simulink model "flamingo_link"  (R2019a)
settings: Solver=FixedStepDiscrete  StartTime=0.0  StopTime=inf  FixedStep=1/500  RelTol=1e-3
PreLoadFcn:
  | x_setpoint_NED = 0;
  | y_setpoint_NED = 0;
  | z_setpoint_NED = 0;
  | vx_setpoint_NED = 0;
  | vy_setpoint_NED = 0;
  | vz_setpoint_NED = 0;
  | afx_setpoint_NED = 0;
  | afy_setpoint_NED = 0;
  | afz_setpoint_NED = 0;
  | yaw_setpoint_NED = 0;
  | yawrate_setpoint_NED = 0;
  | selected_mission = 0;
  | reboot_cmd = 0;
  | return_com = 0;
  | takeoff_com = 0;
  | mission_com = 0;
  | hold_com = 0;
  | land_com = 0;
  | direct_com = 0;
  | origin_com = 0;
InitFcn:
  | x_setpoint_NED = 0;
  | y_setpoint_NED = 0;
  | z_setpoint_NED = 0;
  | vx_setpoint_NED = 0;
  | vy_setpoint_NED = 0;
  | vz_setpoint_NED = 0;
  | afx_setpoint_NED = 0;
  | afy_setpoint_NED = 0;
  | afz_setpoint_NED = 0;
  | yaw_setpoint_NED = 0;
  | yawrate_setpoint_NED = 0;
  | selected_mission = 0;
  | reboot_cmd = 0;
  | return_com = 0;
  | takeoff_com = 0;
  | mission_com = 0;
  | hold_com = 0;
  | land_com = 0;
  | direct_com = 0;
  | origin_com = 0;
undefined symbols (not defined in the file or in its folder): afx, afy, afz, command, confirmation, coordinate_frame, f, Object1, Object2, origin_pos, param1, param2, param3, param4, param5, param6, param7, pitch, roll, Standard_Devices, target_component, target_system, time_boot_ms, time_usec, type_mask, UDP_Protocol, vx, vy, vz, x, y, yaw, yaw_rate, z
libraries: simulink x11, sldrtlib x4, instrumentlib x1
settings Model: Creator=Admin  LastModifiedBy=viconadmin
settings SolverCC: PositivePriorityOrder=on  AutoInsertRateTranBlk=on  InsertRTBMode=Never (minimum delay)
settings DebuggingCC: ReadBeforeWriteMsg=DisableAll  WriteAfterWriteMsg=DisableAll  WriteAfterReadMsg=DisableAll  MultiTaskDSMMsg=none  ArithmeticOperatorsInVariantConditions=warning
settings ModelReferenceCC: UpdateModelReferenceTargets=IfOutOfDate
settings SFSimCC: SFSimEcho=off  SimUseLocalCustomCode=off
settings RTWCC: SystemTargetFile=sldrt.tlc  TemplateMakefile=sldrt.tmf  Description=Simulink Desktop Real-Time  RTWUseLocalCustomCode=off  RTWCompilerOptimization=on
settings CodeAppCC: MaxIdLength=95  StateflowObjectComments=on
settings SimulinkDesktopRealTimeCC: TargetPreCompLibLocation=C:\Program Files\MATLAB\R2019a\toolbox\sldrt\lib\win64  PreserveStateflowLocalDataDimensions=off

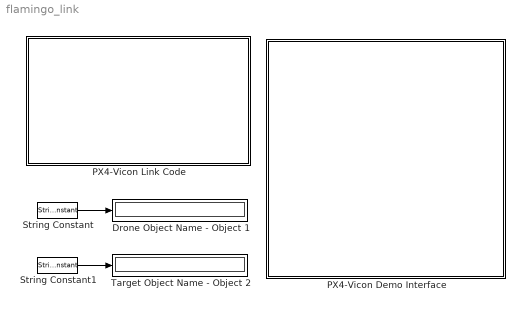
== system flamingo_link ==
  Drone Object Name - Object 1 : Display
  PX4-Vicon Demo Interface : Subsystem
  PX4-Vicon Link Code : Subsystem
  String Constant : StringConstant  String=Object1
  String Constant1 : StringConstant  String=Object2
  Target Object Name - Object 2 : Display
  wires:
  String Constant/1 -> Drone Object Name - Object 1/1
  String Constant1/1 -> Target Object Name - Object 2/1

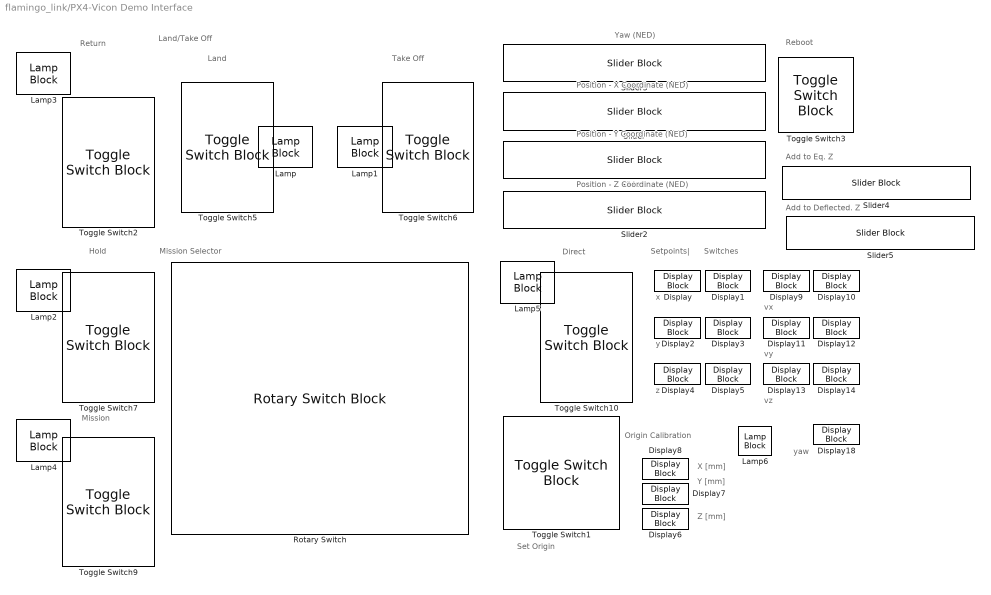
== system flamingo_link/PX4-Vicon Demo Interface ==
  note: Position - X Coordinate (NED)
  note: Position - Y Coordinate (NED)
  note: Position - Z Coordinate (NED)
  note: Yaw (NED)
  note: Mission Selector
  note: Setpoints|
  note: Switches
  note: x
  note: y
  note: z
  note: yaw
  note: Mission
  note: Direct
  note: Hold
  note: Return
  note: Take Off
  note: Land
  note: Land/Take Off
  note: Set Origin
  note: X [mm]
  note: Y [mm]
  note: Z [mm]
  note: Origin Calibration
  note: Reboot
  note: vz
  note: vx
  note: vy
  note: Add to Eq. Z
  note: Add to Deflected. Z
  Display{,1..14,18} (16 alike) : DisplayBlock  LabelPosition=Hide  Format=short
  Lamp{,1..6} (7 alike) : LampBlock  LabelPosition=Hide
  Rotary Switch : RotarySwitchBlock  LabelPosition=Hide
      settings: Values={{'Hold Origin', 'Pulses X', 'Circle'}, [0 1 2]}
  Slider : SliderBlock  LabelPosition=Hide  ScaleMin=-0.5  ScaleMax=0.5  TickInterval=0.10000000000000001
  Slider1 : SliderBlock  LabelPosition=Hide  ScaleMin=-0.5  ScaleMax=0.5  TickInterval=0.10000000000000001
  Slider2 : SliderBlock  LabelPosition=Hide  ScaleMin=-1.5  ScaleMax=0  TickInterval=0.10000000000000001
  Slider3 : SliderBlock  LabelPosition=Hide  ScaleMin=-3  ScaleMax=3
  Slider4 : SliderBlock  LabelPosition=Hide  ScaleMin=-0.14999999999999999  ScaleMax=0.14999999999999999
  Slider5 : SliderBlock  LabelPosition=Hide  ScaleMin=-0.14999999999999999  ScaleMax=0.14999999999999999
  Toggle Switch{1..3,5..7,9..10} (8 alike) : ToggleSwitchBlock  LabelPosition=Hide

== system flamingo_link/PX4-Vicon Link Code ==
  note: MAVLink PX4 Interface Telemetry
  note: MAVLink PX4 Interface Motion Capture
  Data Manipulation : Subsystem
  Decode PX4  Telemetry Data - MAVLink : S-Function  FunctionName=sfun_decode_mavlink  SFunctionDeploymentMode=off  EnableBusSupport=off
  Mavlink Encoded - UDP Packet Output : sldrtlib/Packet Output  SampleTime=1/50  MaxMissedTicks=inf  ShowMissedTicks=off  YieldWhenWaiting=off  DrvName=Standard_Devices/UDP_Protocol  DrvAddress=14551  DrvOptions=[0 14556 48 46 48 46 48 46 48 0 0 0 0 0 0 0 0 0 0 0 0 0 0 0 0 0 0 0 0 0 0 0 0 0 0 0 0 0 0 0 0 0 0 0 0 0 0 0 0 0 0 0 0 0 0 0 0 0 0 0 0 0 0 0 0 0 0 0 0 0 0 0 0 0 0 0 0 0 0 0 0 0 0 0 0 0 0 0 0 0 0 0 0 0 0 0 0 0 0 0 0 0 0 0 0 0 0 0 0 0 0 0 0 0 0 0 0 0 0 0 0 0 0 0 0 0 0 0 0 0 0 0 0 0 0 0 0 0 0 0 0 0 0 0 0 0 0 0 0 0 0 0 0 0 0 0 0 0 0 0 0 0 0 0 0 0 0 0 0 0 0 0 0 0 0 0 0 0 0 0 0 0 0 0 0 0 0 0 0 0 0 0 0 0 0 0 0 0 0 0 0 0 0 0 0 0 0 0 0 0 0 0 0 0 0 0 0 0 0 0 0 0 0 0 0 0 0 0 0 0 0 0 0 0 0 0 0 0 0 0 0 0 0 0 0 0 0 0 0 0 0 0 0 0 0 0]  PacketSize=65  DataTypes='65*uint8'  ShowReady=off  ShowError=off  PacketID=1  ByteOrder=1  InitialValue=[]  FinalValue=[]
      settings: AttributesFormatString=UDP Protocol [14551]  SourceProductName=Simulink Desktop Real-Time
  Mavlink Encoded - UDP Packet Output1 : sldrtlib/Packet Output  Priority=10  SampleTime=1/50  MaxMissedTicks=inf  ShowMissedTicks=off  YieldWhenWaiting=off  DrvName=Standard_Devices/UDP_Protocol  DrvAddress=14551  DrvOptions=[0 14556 48 46 48 46 48 46 48 0 0 0 0 0 0 0 0 0 0 0 0 0 0 0 0 0 0 0 0 0 0 0 0 0 0 0 0 0 0 0 0 0 0 0 0 0 0 0 0 0 0 0 0 0 0 0 0 0 0 0 0 0 0 0 0 0 0 0 0 0 0 0 0 0 0 0 0 0 0 0 0 0 0 0 0 0 0 0 0 0 0 0 0 0 0 0 0 0 0 0 0 0 0 0 0 0 0 0 0 0 0 0 0 0 0 0 0 0 0 0 0 0 0 0 0 0 0 0 0 0 0 0 0 0 0 0 0 0 0 0 0 0 0 0 0 0 0 0 0 0 0 0 0 0 0 0 0 0 0 0 0 0 0 0 0 0 0 0 0 0 0 0 0 0 0 0 0 0 0 0 0 0 0 0 0 0 0 0 0 0 0 0 0 0 0 0 0 0 0 0 0 0 0 0 0 0 0 0 0 0 0 0 0 0 0 0 0 0 0 0 0 0 0 0 0 0 0 0 0 0 0 0 0 0 0 0 0 0 0 0 0 0 0 0 0 0 0 0 0 0 0 0 0 0 0 0]  PacketSize=44  DataTypes='44*uint8'  ShowReady=off  ShowError=off  PacketID=1  ByteOrder=1  InitialValue=[]  FinalValue=[]
      settings: AttributesFormatString=UDP Protocol [14551]  SourceProductName=Simulink Desktop Real-Time
  Mavlink Encoded - UDP Packet Output2 : sldrtlib/Packet Output  SampleTime=1/5  MaxMissedTicks=inf  ShowMissedTicks=off  YieldWhenWaiting=off  DrvName=Standard_Devices/UDP_Protocol  DrvAddress=14551  DrvOptions=[0 14556 48 46 48 46 48 46 48 0 0 0 0 0 0 0 0 0 0 0 0 0 0 0 0 0 0 0 0 0 0 0 0 0 0 0 0 0 0 0 0 0 0 0 0 0 0 0 0 0 0 0 0 0 0 0 0 0 0 0 0 0 0 0 0 0 0 0 0 0 0 0 0 0 0 0 0 0 0 0 0 0 0 0 0 0 0 0 0 0 0 0 0 0 0 0 0 0 0 0 0 0 0 0 0 0 0 0 0 0 0 0 0 0 0 0 0 0 0 0 0 0 0 0 0 0 0 0 0 0 0 0 0 0 0 0 0 0 0 0 0 0 0 0 0 0 0 0 0 0 0 0 0 0 0 0 0 0 0 0 0 0 0 0 0 0 0 0 0 0 0 0 0 0 0 0 0 0 0 0 0 0 0 0 0 0 0 0 0 0 0 0 0 0 0 0 0 0 0 0 0 0 0 0 0 0 0 0 0 0 0 0 0 0 0 0 0 0 0 0 0 0 0 0 0 0 0 0 0 0 0 0 0 0 0 0 0 0 0 0 0 0 0 0 0 0 0 0 0 0 0 0 0 0 0 0]  PacketSize=45  DataTypes='45*uint8'  ShowReady=off  ShowError=off  PacketID=1  ByteOrder=1  InitialValue=[]  FinalValue=[]
      settings: AttributesFormatString=UDP Protocol [14551]  SourceProductName=Simulink Desktop Real-Time
  Packet Input : sldrtlib/Packet Input  SampleTime=1/50  MaxMissedTicks=inf  ShowMissedTicks=off  YieldWhenWaiting=off  DrvName=Standard_Devices/UDP_Protocol  DrvAddress=14551  DrvOptions=[0 14556 48 46 48 46 48 46 48 0 0 0 0 0 0 0 0 0 0 0 0 0 0 0 0 0 0 0 0 0 0 0 0 0 0 0 0 0 0 0 0 0 0 0 0 0 0 0 0 0 0 0 0 0 0 0 0 0 0 0 0 0 0 0 0 0 0 0 0 0 0 0 0 0 0 0 0 0 0 0 0 0 0 0 0 0 0 0 0 0 0 0 0 0 0 0 0 0 0 0 0 0 0 0 0 0 0 0 0 0 0 0 0 0 0 0 0 0 0 0 0 0 0 0 0 0 0 0 0 0 0 0 0 0 0 0 0 0 0 0 0 0 0 0 0 0 0 0 0 0 0 0 0 0 0 0 0 0 0 0 0 0 0 0 0 0 0 0 0 0 0 0 0 0 0 0 0 0 0 0 0 0 0 0 0 0 0 0 0 0 0 0 0 0 0 0 0 0 0 0 0 0 0 0 0 0 0 0 0 0 0 0 0 0 0 0 0 0 0 0 0 0 0 0 0 0 0 0 0 0 0 0 0 0 0 0 0 0 0 0 0 0 0 0 0 0 0 0 0 0 0 0 0 0 0 0]  PacketSize=280  DataTypes='280*uint8'  ShowReady=off  ShowError=off  PacketID=1  ByteOrder=1  ShowTimestamp=off
      settings: AttributesFormatString=UDP Protocol [14551]  SourceProductName=Simulink Desktop Real-Time
  Rate Transition : RateTransition
  Rate Transition1 : RateTransition
  Rate Transition2 : RateTransition
  Vicon Stream - UDP Packet Receive : instrumentlib/UDP Receive  Priority=10  Host=localhost  Port=9090  LocalPort=51001  EnablePortSharing=off  GetLatestData=off  DataSize=256  DataType=uint8  ASCIIFormatting=%f,  Terminator=LF  ByteOrder=BigEndian  EnableBlockingMode=off  Timeout=inf  SampleTime=-1  LocalAddress=0.0.0.0
      settings: SourceProductName=Instrument Control Toolbox
  Visualize Telemetry Data : Subsystem
  wires:
  Rate Transition/1 -> Mavlink Encoded - UDP Packet Output/1
  Packet Input/1 -> Decode PX4  Telemetry Data - MAVLink/1
  Vicon Stream - UDP Packet Receive/1 -> Data Manipulation/1(vicon_data_input)
  Vicon Stream - UDP Packet Receive/2 -> Data Manipulation/2(status)
  Decode PX4  Telemetry Data - MAVLink/2 -> Visualize Telemetry Data/2(telemetry_attitude)
  Data Manipulation/2(Encoded_Mocap_Output) -> Rate Transition1/1
  Decode PX4  Telemetry Data - MAVLink/1 -> Visualize Telemetry Data/1(msg_heartbeat)
  Visualize Telemetry Data/1(FLAG_ARMED) -> Data Manipulation/3(FLAG_ARMED)
  Data Manipulation/1(Encoded_Setpoints_Output) -> Rate Transition/1
  Data Manipulation/3(Encoded_Reboot_Output) -> Rate Transition2/1
  Rate Transition1/1 -> Mavlink Encoded - UDP Packet Output1/1
  Rate Transition2/1 -> Mavlink Encoded - UDP Packet Output2/1

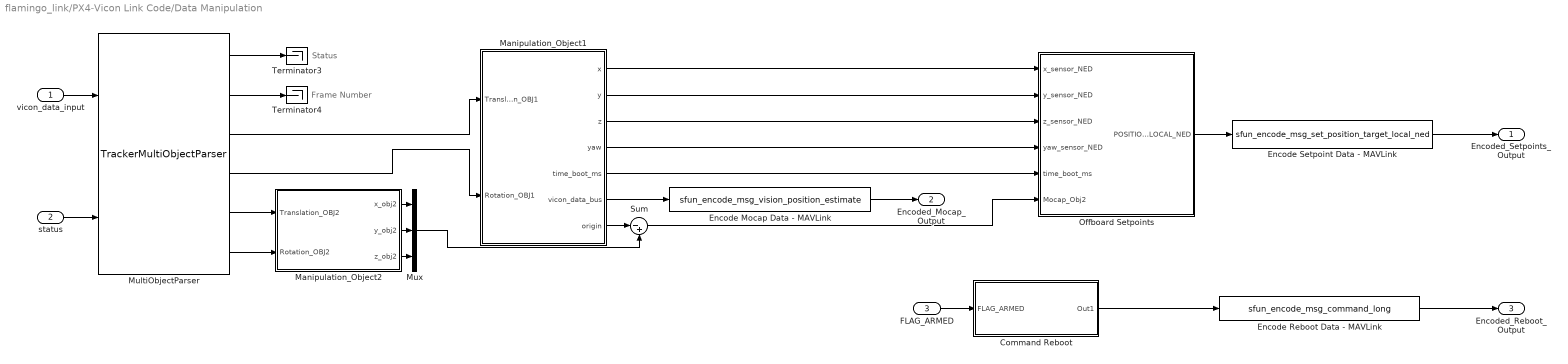
== system flamingo_link/PX4-Vicon Link Code/Data Manipulation ==
  note: Status
  note: Frame Number
  vicon_data_input : Inport
  status : Inport  Port=2
  FLAG_ARMED : Inport  Port=3
  Command Reboot : Subsystem
  "Encode Mocap Data - MAVLink " : S-Function  Priority=10  FunctionName=sfun_encode_msg_vision_position_estimate  SFunctionDeploymentMode=off  EnableBusSupport=off
  Encode Reboot Data - MAVLink : S-Function  FunctionName=sfun_encode_msg_command_long  SFunctionDeploymentMode=off  EnableBusSupport=off
  Encode Setpoint Data - MAVLink : S-Function  FunctionName=sfun_encode_msg_set_position_target_local_ned  SFunctionDeploymentMode=off  EnableBusSupport=off
  Manipulation_Object1 : Subsystem  Priority=10
  Manipulation_Object2 : Subsystem
  MultiObjectParser : S-Function  Tag=Data_Parser_Multi  Priority=10  FunctionName=TrackerMultiObjectParser  Parameters=Object1,Object2  SFunctionModules=TrackerMultiObjectParser  SFunctionDeploymentMode=off  EnableBusSupport=off
      settings: AttributesFormatString=Data_Parser_Multi
  Mux : Mux  Inputs=3
  Offboard Setpoints : Subsystem
  Sum : Sum  Inputs=|-+
  Terminator3 : Terminator
  Terminator4 : Terminator
  Encoded_Setpoints_Output : Outport
  Encoded_Mocap_Output : Outport  Port=2
  Encoded_Reboot_Output : Outport  Port=3
  wires:
  MultiObjectParser/3 -> Manipulation_Object1/1(Translation_OBJ1)
  MultiObjectParser/2 -> Terminator4/1
  Manipulation_Object1/1(x) -> Offboard Setpoints/1(x_sensor_NED)
  MultiObjectParser/1 -> Terminator3/1
  Manipulation_Object1/6(vicon_data_bus) -> "Encode Mocap Data - MAVLink "/1
  MultiObjectParser/5 -> Manipulation_Object2/1(Translation_OBJ2)
  MultiObjectParser/6 -> Manipulation_Object2/2(Rotation_OBJ2)
  MultiObjectParser/4 -> Manipulation_Object1/2(Rotation_OBJ1)
  Manipulation_Object1/4(yaw) -> Offboard Setpoints/4(yaw_sensor_NED)
  status/1 -> MultiObjectParser/2
  Manipulation_Object1/3(z) -> Offboard Setpoints/3(z_sensor_NED)
  Manipulation_Object1/2(y) -> Offboard Setpoints/2(y_sensor_NED)
  "Encode Mocap Data - MAVLink "/1 -> Encoded_Mocap_Output/1
  vicon_data_input/1 -> MultiObjectParser/1
  Manipulation_Object1/5(time_boot_ms) -> Offboard Setpoints/5(time_boot_ms)
  Offboard Setpoints/1(POSITION_TARGET_LOCAL_NED) -> Encode Setpoint Data - MAVLink/1
  Encode Setpoint Data - MAVLink/1 -> Encoded_Setpoints_Output/1
  Mux/1 -> Sum/2
  Command Reboot/1(Out1) -> Encode Reboot Data - MAVLink/1
  FLAG_ARMED/1 -> Command Reboot/1(FLAG_ARMED)
  Encode Reboot Data - MAVLink/1 -> Encoded_Reboot_Output/1
  Manipulation_Object2/3(z_obj2) -> Mux/3
  Manipulation_Object2/2(y_obj2) -> Mux/2
  Manipulation_Object2/1(x_obj2) -> Mux/1
  Manipulation_Object1/7(origin) -> Sum/1
  Sum/1 -> Offboard Setpoints/6(Mocap_Obj2)

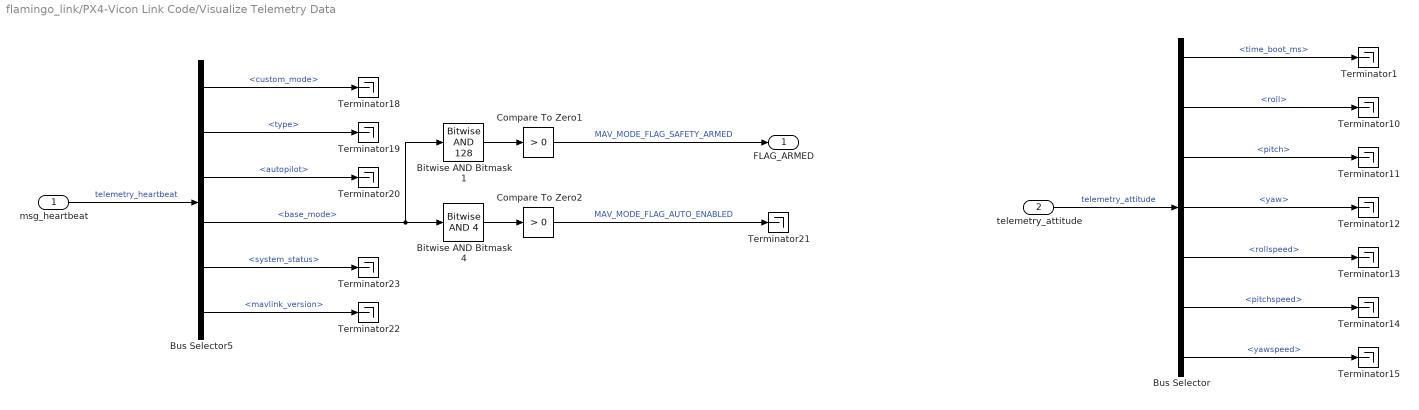
== system flamingo_link/PX4-Vicon Link Code/Visualize Telemetry Data ==
  msg_heartbeat : Inport
  telemetry_attitude : Inport  Port=2
  Bitwise AND Bitmask 1 : simulink/Logic and Bit Operations/Bitwise Operator  logicop=AND  UseBitMask=on  BitMask=128  BitMaskRealWorld=Stored Integer
  Bitwise AND Bitmask 4 : simulink/Logic and Bit Operations/Bitwise Operator  logicop=AND  UseBitMask=on  BitMask=4  BitMaskRealWorld=Stored Integer
  Bus Selector : BusSelector  OutputSignals=time_boot_ms,roll,pitch,yaw,rollspeed,pitchspeed,yawspeed
  Bus Selector5 : BusSelector  OutputSignals=custom_mode,type,autopilot,base_mode,system_status,mavlink_version
  Compare To Zero1 : simulink/Logic and Bit Operations/Compare To Zero  relop=>  OutDataTypeStr=boolean
  Compare To Zero2 : simulink/Logic and Bit Operations/Compare To Zero  relop=>  OutDataTypeStr=boolean
  Terminator{1,10..15,18..23} (13 alike) : Terminator
  FLAG_ARMED : Outport
  wires:
  Bus Selector/7 -> Terminator15/1  "<yawspeed>"
  Bus Selector/5 -> Terminator13/1  "<rollspeed>"
  Bus Selector/2 -> Terminator10/1  "<roll>"
  Bus Selector/1 -> Terminator1/1  "<time_boot_ms>"
  Bus Selector/4 -> Terminator12/1  "<yaw>"
  Bus Selector/3 -> Terminator11/1  "<pitch>"
  Bus Selector/6 -> Terminator14/1  "<pitchspeed>"
  telemetry_attitude/1 -> Bus Selector/1  "telemetry_attitude"
  Bus Selector5/4 -> Bitwise AND Bitmask 1/1, Bitwise AND Bitmask 4/1  "<base_mode>"
  Bitwise AND Bitmask 4/1 -> Compare To Zero2/1
  Bitwise AND Bitmask 1/1 -> Compare To Zero1/1
  Bus Selector5/3 -> Terminator20/1  "<autopilot>"
  Compare To Zero1/1 -> FLAG_ARMED/1  "MAV_MODE_FLAG_SAFETY_ARMED"
  Bus Selector5/6 -> Terminator22/1  "<mavlink_version>"
  Bus Selector5/5 -> Terminator23/1  "<system_status>"
  Bus Selector5/2 -> Terminator19/1  "<type>"
  Bus Selector5/1 -> Terminator18/1  "<custom_mode>"
  msg_heartbeat/1 -> Bus Selector5/1  "telemetry_heartbeat"
  Compare To Zero2/1 -> Terminator21/1  "MAV_MODE_FLAG_AUTO_ENABLED"

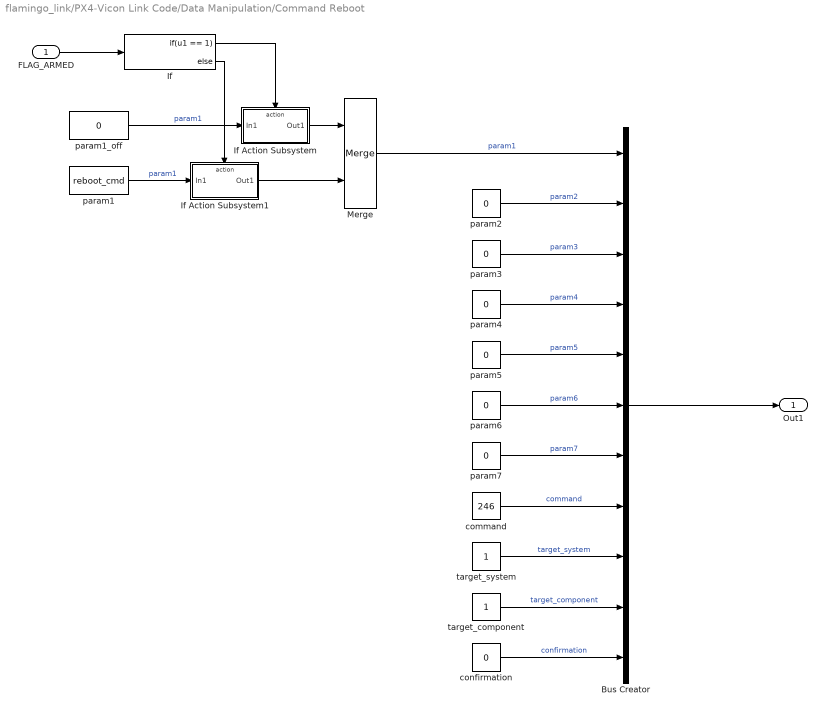
== system flamingo_link/PX4-Vicon Link Code/Data Manipulation/Command Reboot ==
  FLAG_ARMED : Inport
  Bus Creator : BusCreator  Inputs=param1,param2,param3,param4,param5,param6,param7,command,target_system,target_component,confirmation  OutDataTypeStr=Bus: mavlink_command_long_t
  If : If  IfExpression=u1 == 1
  If Action Subsystem : Subsystem  TreatAsAtomicUnit=on
  If Action Subsystem1 : Subsystem  TreatAsAtomicUnit=on
  Merge : Merge
  command : Constant  Value=246  OutDataTypeStr=uint16
  confirmation : Constant  Value=0  OutDataTypeStr=uint8
  param1 : Constant  Value=reboot_cmd  OutDataTypeStr=single
  param1_off : Constant  Value=0  OutDataTypeStr=single
  param{2..7} (6 alike) : Constant  Value=0  OutDataTypeStr=single
  target_component : Constant  OutDataTypeStr=uint8
  target_system : Constant  OutDataTypeStr=uint8
  Out1 : Outport
  wires:
  Bus Creator/1 -> Out1/1
  Merge/1 -> Bus Creator/1  "param1"
  param2/1 -> Bus Creator/2  "param2"
  param3/1 -> Bus Creator/3  "param3"
  param4/1 -> Bus Creator/4  "param4"
  command/1 -> Bus Creator/8  "command"
  target_system/1 -> Bus Creator/9  "target_system"
  target_component/1 -> Bus Creator/10  "target_component"
  param5/1 -> Bus Creator/5  "param5"
  param6/1 -> Bus Creator/6  "param6"
  param7/1 -> Bus Creator/7  "param7"
  confirmation/1 -> Bus Creator/11  "confirmation"
  FLAG_ARMED/1 -> If/1
  If/1 -> If Action Subsystem/Action
  If/2 -> If Action Subsystem1/Action
  param1/1 -> If Action Subsystem1/1(In1)  "param1"
  param1_off/1 -> If Action Subsystem/1(In1)  "param1"
  If Action Subsystem1/1(Out1) -> Merge/2
  If Action Subsystem/1(Out1) -> Merge/1

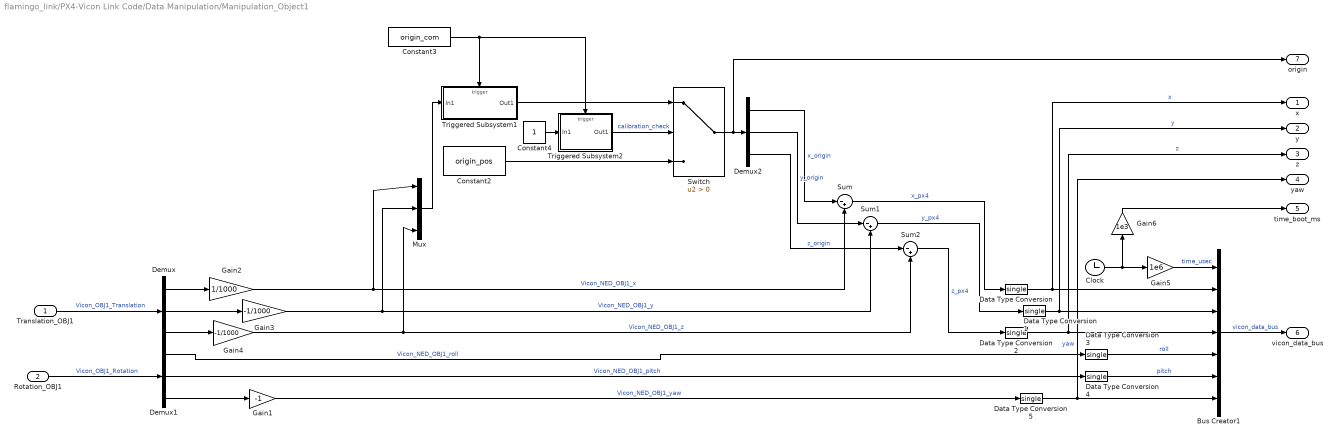
== system flamingo_link/PX4-Vicon Link Code/Data Manipulation/Manipulation_Object1 ==
  Translation_OBJ1 : Inport
  Rotation_OBJ1 : Inport  Port=2
  Bus Creator1 : BusCreator  Inputs=time_usec,x,y,z,roll,pitch,yaw  OutDataTypeStr=Bus: mavlink_vision_position_estimate_t
  Clock : Clock
  Constant2 : Constant  Value=origin_pos
  Constant3 : Constant  Value=origin_com
  Constant4 : Constant
  Data Type Conversion{,1..5} (6 alike) : DataTypeConversion  OutDataTypeStr=single
  Demux : Demux  Outputs=3
  Demux1 : Demux  Outputs=3
  Demux2 : Demux  Outputs=3
  Gain1 : Gain  Gain=-1  OutDataTypeStr=Inherit: Same as input
  Gain2 : Gain  Gain=1/1000  OutDataTypeStr=double
  Gain3 : Gain  Gain=-1/1000  OutDataTypeStr=double
  Gain4 : Gain  Gain=-1/1000  OutDataTypeStr=double
  Gain5 : Gain  Gain=1e6  OutDataTypeStr=double
  Gain6 : Gain  Gain=1e3  OutDataTypeStr=double
  Mux : Mux  Inputs=3
  Sum : Sum  Inputs=|-+
  Sum1 : Sum  Inputs=|-+
  Sum2 : Sum  Inputs=|-+
  Switch : Switch  Criteria=u2 > Threshold
  Triggered Subsystem1 : Subsystem  TreatAsAtomicUnit=on
  Triggered Subsystem2 : Subsystem  TreatAsAtomicUnit=on
  x : Outport
  y : Outport  Port=2
  z : Outport  Port=3
  yaw : Outport  Port=4
  time_boot_ms : Outport  Port=5
  vicon_data_bus : Outport  Port=6
  origin : Outport  Port=7
  wires:
  Data Type Conversion1/1 -> y/1, Bus Creator1/3  "y"
  Bus Creator1/1 -> vicon_data_bus/1  "vicon_data_bus"
  Data Type Conversion5/1 -> yaw/1, Bus Creator1/7  "yaw"
  Gain4/1 -> Mux/3, Sum2/2  "Vicon_NED_OBJ1_z"
  Gain1/1 -> Data Type Conversion5/1  "Vicon_NED_OBJ1_yaw"
  Data Type Conversion4/1 -> Bus Creator1/6  "pitch"
  Gain2/1 -> Mux/1, Sum/2  "Vicon_NED_OBJ1_x"
  Gain3/1 -> Mux/2, Sum1/2  "Vicon_NED_OBJ1_y"
  Demux/3 -> Gain4/1
  Data Type Conversion2/1 -> z/1, Bus Creator1/4  "z"
  Gain5/1 -> Bus Creator1/1  "time_usec"
  Demux1/2 -> Data Type Conversion4/1  "Vicon_NED_OBJ1_pitch"
  Data Type Conversion/1 -> x/1, Bus Creator1/2  "x"
  Data Type Conversion3/1 -> Bus Creator1/5  "roll"
  Demux1/1 -> Data Type Conversion3/1  "Vicon_NED_OBJ1_roll"
  Clock/1 -> Gain5/1, Gain6/1
  Demux1/3 -> Gain1/1
  Gain6/1 -> time_boot_ms/1
  Demux/2 -> Gain3/1
  Demux/1 -> Gain2/1
  Translation_OBJ1/1 -> Demux/1  "Vicon_OBJ1_Translation"
  Rotation_OBJ1/1 -> Demux1/1  "Vicon_OBJ1_Rotation"
  Switch/1 -> origin/1, Demux2/1
  Triggered Subsystem1/1(Out1) -> Switch/1
  Constant2/1 -> Switch/3
  Demux2/3 -> Sum2/1  "z_origin"
  Demux2/1 -> Sum/1  "x_origin"
  Triggered Subsystem2/1(Out1) -> Switch/2  "calibration_check"
  Constant3/1 -> Triggered Subsystem1/Trigger, Triggered Subsystem2/Trigger
  Constant4/1 -> Triggered Subsystem2/1(In1)
  Demux2/2 -> Sum1/1  "y_origin"
  Mux/1 -> Triggered Subsystem1/1(In1)
  Sum/1 -> Data Type Conversion/1  "x_px4"
  Sum1/1 -> Data Type Conversion1/1  "y_px4"
  Sum2/1 -> Data Type Conversion2/1  "z_px4"

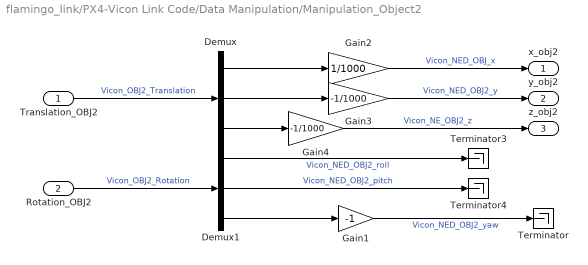
== system flamingo_link/PX4-Vicon Link Code/Data Manipulation/Manipulation_Object2 ==
  Translation_OBJ2 : Inport
  Rotation_OBJ2 : Inport  Port=2
  Demux : Demux  Outputs=3
  Demux1 : Demux  Outputs=3
  Gain1 : Gain  Gain=-1  OutDataTypeStr=Inherit: Same as input
  Gain2 : Gain  Gain=1/1000  OutDataTypeStr=double
  Gain3 : Gain  Gain=-1/1000  OutDataTypeStr=double
  Gain4 : Gain  Gain=-1/1000  OutDataTypeStr=double
  Terminator : Terminator
  Terminator3 : Terminator
  Terminator4 : Terminator
  x_obj2 : Outport  VectorParamsAs1DForOutWhenUnconnected=on
  y_obj2 : Outport  Port=2  VectorParamsAs1DForOutWhenUnconnected=on
  z_obj2 : Outport  Port=3  VectorParamsAs1DForOutWhenUnconnected=on
  wires:
  Demux1/2 -> Terminator4/1  "Vicon_NED_OBJ2_pitch"
  Demux/3 -> Gain4/1
  Demux1/1 -> Terminator3/1  "Vicon_NED_OBJ2_roll"
  Demux1/3 -> Gain1/1
  Demux/2 -> Gain3/1
  Translation_OBJ2/1 -> Demux/1  "Vicon_OBJ2_Translation"
  Rotation_OBJ2/1 -> Demux1/1  "Vicon_OBJ2_Rotation"
  Demux/1 -> Gain2/1
  Gain3/1 -> y_obj2/1  "Vicon_NED_OBJ2_y"
  Gain4/1 -> z_obj2/1  "Vicon_NE_OBJ2_z"
  Gain2/1 -> x_obj2/1  "Vicon_NED_OBJ_x"
  Gain1/1 -> Terminator/1  "Vicon_NED_OBJ2_yaw"

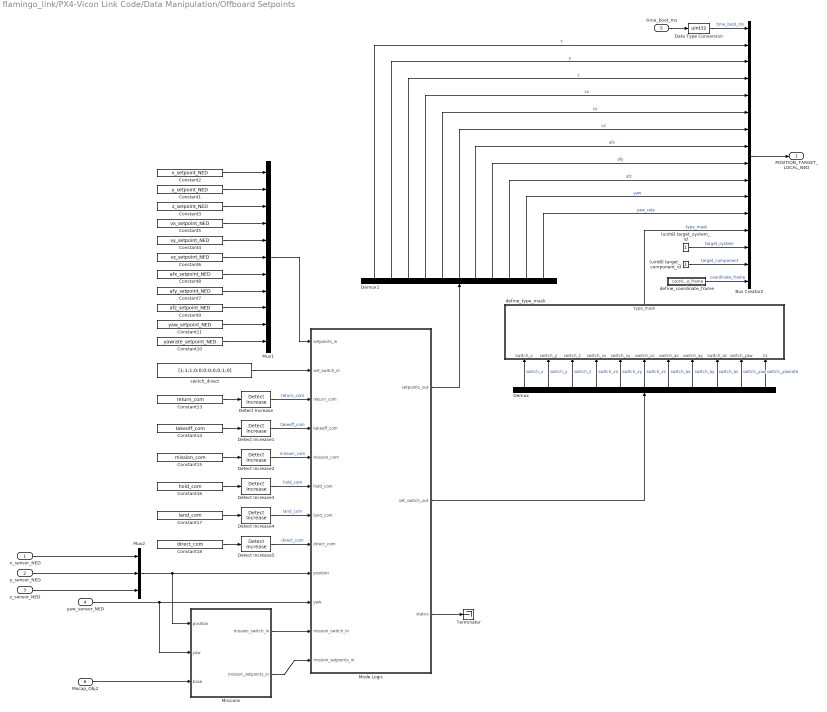
== system flamingo_link/PX4-Vicon Link Code/Data Manipulation/Offboard Setpoints ==
  x_sensor_NED : Inport
  y_sensor_NED : Inport  Port=2
  z_sensor_NED : Inport  Port=3
  yaw_sensor_NED : Inport  Port=4
  time_boot_ms : Inport  Port=5
  Mocap_Obj2 : Inport  Port=6
  (uint8) target_component_id : Constant  OutDataTypeStr=uint8
  (uint8) target_system_id : Constant  OutDataTypeStr=uint8
  Bus Creator2 : BusCreator  Inputs=time_boot_ms,x,y,z,vx,vy,vz,afx,afy,afz,yaw,yaw_rate,type_mask,target_system,target_component,coordinate_frame  OutDataTypeStr=Bus: mavlink_set_position_target_local_ned_t
  Constant1 : Constant  Value=y_setpoint_NED  OutDataTypeStr=single
  Constant10 : Constant  Value=yawrate_setpoint_NED  OutDataTypeStr=single
  Constant11 : Constant  Value=yaw_setpoint_NED  OutDataTypeStr=single
  Constant13 : Constant  Value=return_com  OutDataTypeStr=single
  Constant14 : Constant  Value=takeoff_com  OutDataTypeStr=single
  Constant15 : Constant  Value=mission_com  OutDataTypeStr=single
  Constant16 : Constant  Value=hold_com  OutDataTypeStr=single
  Constant17 : Constant  Value=land_com  OutDataTypeStr=single
  Constant18 : Constant  Value=direct_com  OutDataTypeStr=single
  Constant2 : Constant  Value=x_setpoint_NED  OutDataTypeStr=single
  Constant3 : Constant  Value=z_setpoint_NED  OutDataTypeStr=single
  Constant4 : Constant  Value=vy_setpoint_NED  OutDataTypeStr=single
  Constant5 : Constant  Value=vx_setpoint_NED  OutDataTypeStr=single
  Constant6 : Constant  Value=vz_setpoint_NED  OutDataTypeStr=single
  Constant7 : Constant  Value=afy_setpoint_NED  OutDataTypeStr=single
  Constant8 : Constant  Value=afx_setpoint_NED  OutDataTypeStr=single
  Constant9 : Constant  Value=afz_setpoint_NED  OutDataTypeStr=single
  Data Type Conversion : DataTypeConversion  OutDataTypeStr=uint32
  Demux : Demux  Outputs=11
  Demux1 : Demux  Outputs=11
  Detect Increase{,1..5} (6 alike) : simulink/Logic and Bit Operations/Detect Increase  vinit=0.0  OutDataTypeStr=boolean
  Missions : Subsystem
  Mode Logic : Stateflow chart  BlockKeywords=__PRM__SERIALIZED__DATA__:Stateflow Chart,Stateflow Diagram  TreatAsAtomicUnit=on
  Mux1 : Mux  Inputs=11
  Mux2 : Mux  Inputs=3
  Terminator : Terminator
  define_coordinate_frame : Subsystem
  define_type_mask : Subsystem
  switch_direct : Constant  Value=[1;1;1;0;0;0;0;0;0;1;0]  OutDataTypeStr=single
  POSITION_TARGET_LOCAL_NED : Outport
  wires:
  Bus Creator2/1 -> POSITION_TARGET_LOCAL_NED/1
  time_boot_ms/1 -> Data Type Conversion/1
  define_type_mask/1(type_mask) -> Bus Creator2/13  "type_mask"
  (uint8) target_system_id/1 -> Bus Creator2/14  "target_system"
  (uint8) target_component_id/1 -> Bus Creator2/15  "target_component"
  define_coordinate_frame/1(coordinate_frame) -> Bus Creator2/16  "coordinate_frame"
  Data Type Conversion/1 -> Bus Creator2/1  "time_boot_ms"
  Demux/11 -> define_type_mask/11(switch_yawrate)  "switch_yawrate"
  Demux/10 -> define_type_mask/10(switch_yaw)  "switch_yaw"
  Demux/9 -> define_type_mask/9(switch_az)  "switch_az"
  Demux/8 -> define_type_mask/8(switch_ay)  "switch_ay"
  Demux/7 -> define_type_mask/7(switch_ax)  "switch_ax"
  Demux/6 -> define_type_mask/6(switch_vz)  "switch_vz"
  Demux/5 -> define_type_mask/5(switch_vy)  "switch_vy"
  Demux/4 -> define_type_mask/4(switch_vx)  "switch_vx"
  Demux/3 -> define_type_mask/3(switch_z)  "switch_z"
  Demux/2 -> define_type_mask/2(switch_y)  "switch_y"
  Demux/1 -> define_type_mask/1(switch_x)  "switch_x"
  Mux1/1 -> Mode Logic/1(setpoints_in)
  Constant5/1 -> Mux1/4
  Constant4/1 -> Mux1/5
  Constant6/1 -> Mux1/6
  Constant8/1 -> Mux1/7
  Constant7/1 -> Mux1/8
  Constant9/1 -> Mux1/9
  Constant10/1 -> Mux1/11
  Demux1/11 -> Bus Creator2/12  "yaw_rate"
  Demux1/10 -> Bus Creator2/11  "yaw"
  Demux1/9 -> Bus Creator2/10  "afz"
  Demux1/8 -> Bus Creator2/9  "afy"
  Demux1/7 -> Bus Creator2/8  "afx"
  Demux1/6 -> Bus Creator2/7  "vz"
  Demux1/5 -> Bus Creator2/6  "vy"
  Demux1/4 -> Bus Creator2/5  "vx"
  Demux1/3 -> Bus Creator2/4  "z"
  Demux1/2 -> Bus Creator2/3  "y"
  Demux1/1 -> Bus Creator2/2  "x"
  Mux2/1 -> Missions/1(position), Mode Logic/9(position)
  x_sensor_NED/1 -> Mux2/1
  y_sensor_NED/1 -> Mux2/2
  z_sensor_NED/1 -> Mux2/3
  yaw_sensor_NED/1 -> Missions/2(yaw), Mode Logic/10(yaw)
  Missions/1(mission_switch_in) -> Mode Logic/11(mission_switch_in)
  Missions/2(mission_setpoints_in) -> Mode Logic/12(mission_setpoints_in)
  Mode Logic/3(status) -> Terminator/1
  switch_direct/1 -> Mode Logic/2(set_switch_in)
  Mode Logic/2(set_switch_out) -> Demux/1
  Detect Increase5/1 -> Mode Logic/8(direct_com)  "direct_com"
  Detect Increase/1 -> Mode Logic/3(return_com)  "return_com"
  Detect Increase2/1 -> Mode Logic/5(mission_com)  "mission_com"
  Detect Increase1/1 -> Mode Logic/4(takeoff_com)  "takeoff_com"
  Constant15/1 -> Detect Increase2/1
  Constant18/1 -> Detect Increase5/1
  Detect Increase4/1 -> Mode Logic/7(land_com)  "land_com"
  Constant16/1 -> Detect Increase3/1
  Constant17/1 -> Detect Increase4/1
  Constant14/1 -> Detect Increase1/1
  Detect Increase3/1 -> Mode Logic/6(hold_com)  "hold_com"
  Constant13/1 -> Detect Increase/1
  Constant2/1 -> Mux1/1
  Constant11/1 -> Mux1/10
  Constant3/1 -> Mux1/3
  Constant1/1 -> Mux1/2
  Mocap_Obj2/1 -> Missions/3(base)
  Mode Logic/1(setpoints_out) -> Demux1/1

== system flamingo_link/PX4-Vicon Link Code/Data Manipulation/Command Reboot/If Action Subsystem ==
  In1 : Inport
  Action Port : ActionPort  ActionPortLabel=if(u1 == 1)
  Out1 : Outport
  wires:
  In1/1 -> Out1/1

== system flamingo_link/PX4-Vicon Link Code/Data Manipulation/Command Reboot/If Action Subsystem1 ==
  In1 : Inport
  Action Port : ActionPort  ActionPortLabel=else
  Out1 : Outport
  wires:
  In1/1 -> Out1/1

== system flamingo_link/PX4-Vicon Link Code/Data Manipulation/Manipulation_Object1/Triggered Subsystem1 ==
  In1 : Inport
  Trigger : TriggerPort  VariantControl=Variant  InitialTriggerSignalState=zero
  Out1 : Outport  VectorParamsAs1DForOutWhenUnconnected=on
  wires:
  In1/1 -> Out1/1

== system flamingo_link/PX4-Vicon Link Code/Data Manipulation/Manipulation_Object1/Triggered Subsystem2 ==
  In1 : Inport
  Trigger : TriggerPort  VariantControl=Variant  InitialTriggerSignalState=zero
  Out1 : Outport  VectorParamsAs1DForOutWhenUnconnected=on
  wires:
  In1/1 -> Out1/1

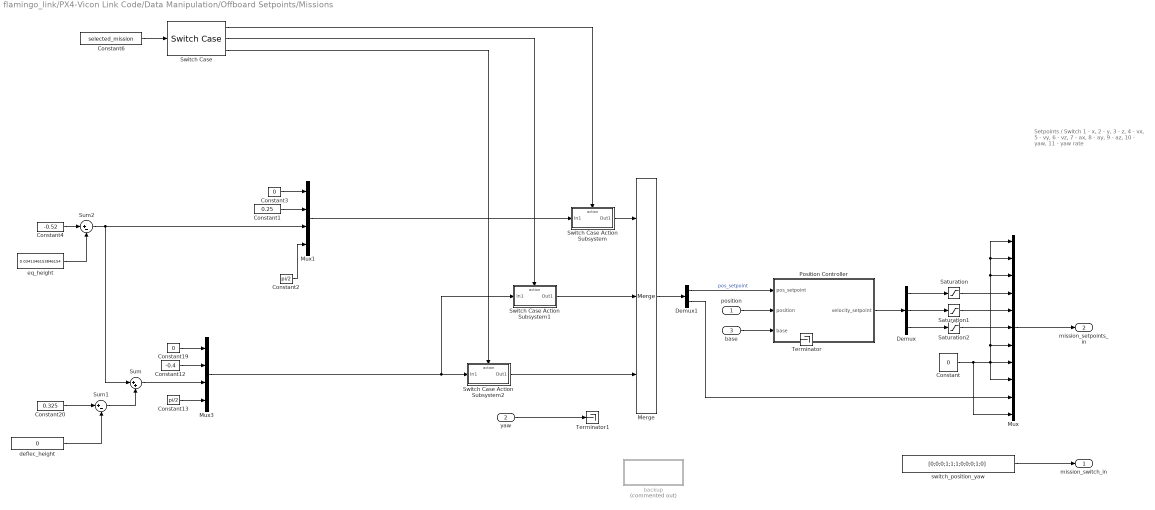
== system flamingo_link/PX4-Vicon Link Code/Data Manipulation/Offboard Setpoints/Missions ==
  note: Setpoints / Switch
      | 1 - x,
      | 2 - y,
      | 3 - z,
      | 4 - vx,
      | 5 - vy,
      | 6 - vz,
      | 7 - ax,
      | 8 - ay,
      | 9 - az,
      | 10 - yaw,
      | 11 - yaw rate
  position : Inport
  yaw : Inport  Port=2
  base : Inport  Port=3
  Constant : Constant  Value=0  OutDataTypeStr=single
  Constant1 : Constant  Value=0.25  OutDataTypeStr=single
  Constant12 : Constant  Value=-0.4  OutDataTypeStr=single
  Constant13 : Constant  Value=pi/2  OutDataTypeStr=single
  Constant19 : Constant  Value=0  OutDataTypeStr=single
  Constant2 : Constant  Value=pi/2  OutDataTypeStr=single
  Constant20 : Constant  Value=0.325  OutDataTypeStr=single
  Constant3 : Constant  Value=0  OutDataTypeStr=single
  Constant4 : Constant  Value=-0.52  OutDataTypeStr=single
  Constant6 : Constant  Value=selected_mission
  Demux : Demux  Outputs=3
  Demux1 : Demux  Outputs=2
  Merge : Merge  Inputs=3
  Mux : Mux  Inputs=11
  Mux1 : Mux
  Mux3 : Mux
  Position Controller : Subsystem
  Saturation : Saturate  UpperLimit=1  LowerLimit=-1
  Saturation1 : Saturate  UpperLimit=1  LowerLimit=-1
  Saturation2 : Saturate  UpperLimit=1  LowerLimit=-1
  Sum : Sum  Inputs=|++
  Sum1 : Sum  Inputs=|+-
  Sum2 : Sum  Inputs=|+-
  Switch Case : SwitchCase  CaseConditions={0,1,2}  ShowDefaultCase=off
  Switch Case Action Subsystem : Subsystem  TreatAsAtomicUnit=on
  Switch Case Action Subsystem1 : Subsystem  TreatAsAtomicUnit=on
  Switch Case Action Subsystem2 : Subsystem  TreatAsAtomicUnit=on
  Terminator : Terminator
  Terminator1 : Terminator
  backup : Subsystem  Commented=on
  deflec_height : Constant  Value=0  OutDataTypeStr=single
  eq_height : Constant  Value=0.0341346153846154  OutDataTypeStr=single
  switch_position_yaw : Constant  Value=[0;0;0;1;1;1;0;0;0;1;0]  OutDataTypeStr=single
  mission_switch_in : Outport
  mission_setpoints_in : Outport  Port=2
  wires:
  switch_position_yaw/1 -> mission_switch_in/1
  Constant/1 -> Mux/11, Mux/9, Mux/1, Mux/2, Mux/3, Mux/7, Mux/8
  Mux/1 -> mission_setpoints_in/1
  Constant6/1 -> Switch Case/1
  Switch Case/1 -> Switch Case Action Subsystem/Action
  Switch Case/2 -> Switch Case Action Subsystem1/Action
  Switch Case Action Subsystem/1(Out1) -> Merge/1
  Switch Case Action Subsystem1/1(Out1) -> Merge/2
  Merge/1 -> Demux1/1
  Demux/1 -> Saturation/1
  Demux/2 -> Saturation1/1
  Demux/3 -> Saturation2/1
  Saturation/1 -> Mux/4
  Saturation1/1 -> Mux/5
  Saturation2/1 -> Mux/6
  Constant13/1 -> Mux3/4
  Mux3/1 -> Switch Case Action Subsystem1/1(In1), Switch Case Action Subsystem2/1(In1)
  Switch Case/3 -> Switch Case Action Subsystem2/Action
  Switch Case Action Subsystem2/1(Out1) -> Merge/3
  yaw/1 -> Terminator1/1
  Constant12/1 -> Mux3/2
  Constant19/1 -> Mux3/1
  base/1 -> Position Controller/3("base ")
  Demux1/2 -> Mux/10
  Demux1/1 -> Position Controller/1(pos_setpoint)  "pos_setpoint"
  position/1 -> Position Controller/2(position)
  Position Controller/1(velocity_setpoint) -> Demux/1
  Mux1/1 -> Switch Case Action Subsystem/1(In1)
  Constant3/1 -> Mux1/1
  Constant1/1 -> Mux1/2
  Constant2/1 -> Mux1/4
  Sum2/1 -> Mux1/3, Sum/1
  Constant20/1 -> Sum1/1
  Sum/1 -> Mux3/3
  Sum1/1 -> Sum/2
  deflec_height/1 -> Sum1/2
  Constant4/1 -> Sum2/1
  eq_height/1 -> Sum2/2

== system flamingo_link/PX4-Vicon Link Code/Data Manipulation/Offboard Setpoints/define_coordinate_frame ==
  note: uint8_t
      |
      | MAV_FRAME
      | Value Field Name Description
      | 0 MAV_FRAME_GLOBAL Global (WGS84) coordinate frame + MSL altitude. First value / x: latitude, second value / y: longitude, third value / z: positive altitude over mean sea level (MSL).
      | 1 MAV_FRAME_LOCAL_NED Local coordinate frame, Z-down (x: north, y: east, z: down).
      | 2 MAV_FRAME_MISSION NOT a coordinate frame, indicates a mission command.
      | 3 MAV_FRAME_GLOBAL_RELATIVE_ALT Global (WGS84) coordinate frame + altitude relative to the home position. First value / x: latitude, second value / y: longitude, third value / z: positive altitude with 0 being at the altitude of the home location.
      | 4 MAV_FRAME_LOCAL_ENU Local coordinate frame, Z-up (x: east, y: north, z: up).
      | 5 MAV_FRAME_GLOBAL_INT Global (WGS84) coordinate frame (scaled) + MSL altitude. First value / x: latitude in degrees*1.0e-7, second value / y: longitude in degrees*1.0e-7, third value / z: positive altitude over mean sea level (MSL).
      | 6 MAV_FRAME_GLOBAL_RELATIVE_ALT_INT Global (WGS84) coordinate frame (scaled) + altitude relative to the home position. First value / x: latitude in degrees*10e-7, second value / y: longitude in degrees*10e-7, third value / z: positive altitude with 0 being at the altitude of the home location.
      | 7 MAV_FRAME_LOCAL_OFFSET_NED Offset to the current local frame. Anything expressed in this frame should be added to the current local frame position.
      | 8 MAV_FRAME_BODY_NED Setpoint in body NED frame. This makes sense if all position control is externalized - e.g. useful to command 2 m/s^2 acceleration to the right.
      | 9 MAV_FRAME_BODY_OFFSET_NED Offset in body NED frame. This makes sense if adding setpoints to the current flight path, to avoid an obstacle - e.g. useful to command 2 m/s^2 acceleration to the east.
      | 10 MAV_FRAME_GLOBAL_TERRAIN_ALT Global (WGS84) coordinate frame with AGL altitude (at the waypoint coordinate). First value / x: latitude in degrees, second value / y: longitude in degrees, third value / z: positive altitude in meters with 0 being at ground level in terrain model.
      | 11 MAV_FRAME_GLOBAL_TERRAIN_ALT_INT Global (WGS84) coordinate frame (scaled) with AGL altitude (at the waypoint coordinate). First value / x: latitude in degrees*10e-7, second value / y: longitude in degrees*10e-7, third value / z: positive altitude in meters with 0 being at ground level in terrain model.
      | 12 MAV_FRAME_BODY_FRD Body fixed frame of reference, Z-down (x: forward, y: right, z: down).
      | 13 MAV_FRAME_BODY_FLU Body fixed frame of reference, Z-up (x: forward, y: left, z: up).
      | 14 MAV_FRAME_MOCAP_NED Odometry local coordinate frame of data given by a motion capture system, Z-down (x: north, y: east, z: down).
      | 15 MAV_FRAME_MOCAP_ENU Odometry local coordinate frame of data given by a motion capture system, Z-up (x: east, y: north, z: up).
      | 16 MAV_FRAME_VISION_NED Odometry local coordinate frame of data given by a vision estimation system, Z-down (x: north, y: east, z: down).
      | 17 MAV_FRAME_VISION_ENU Odometry local coordinate frame of data given by a vision estimation system, Z-up (x: east, y: north, z: up).
      | 18 MAV_FRAME_ESTIM_NED Odometry local coordinate frame of data given by an estimator running onboard the vehicle, Z-down (x: north, y: east, z: down).
      | 19 MAV_FRAME_ESTIM_ENU Odometry local coordinate frame of data given by an estimator running onboard the vehicle, Z-up (x: east, y: noth, z: up).
  (uint8) MAV_FRAME_LOCAL_NED : Constant  OutDataTypeStr=uint8
  coordinate_frame : Outport
  wires:
  (uint8) MAV_FRAME_LOCAL_NED/1 -> coordinate_frame/1

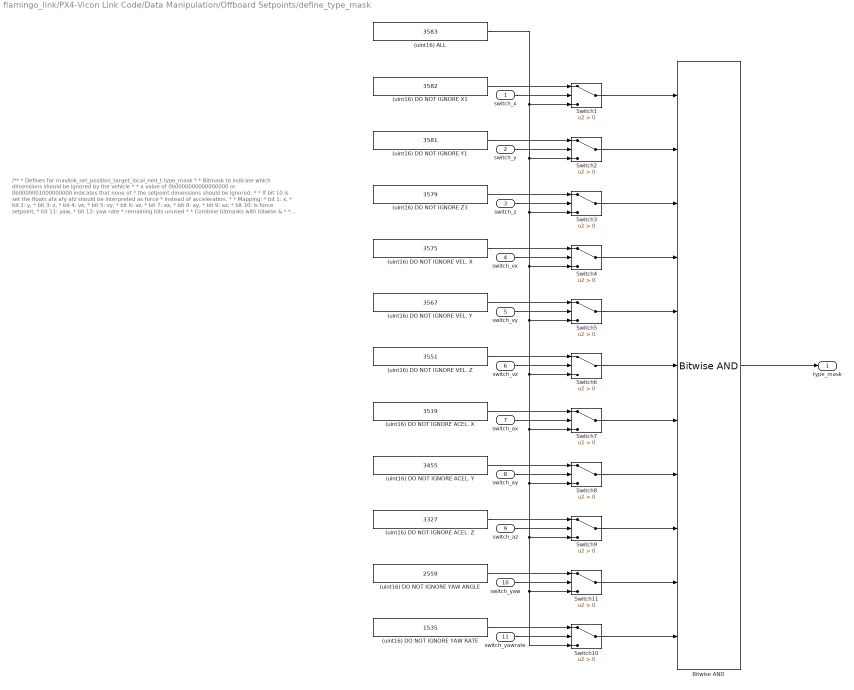
== system flamingo_link/PX4-Vicon Link Code/Data Manipulation/Offboard Setpoints/define_type_mask ==
  note: /**
      |  * Defines for mavlink_set_position_target_local_ned_t.type_mask
      |  *
      |  * Bitmask to indicate which dimensions should be ignored by the vehicle
      |  *
      |  * a value of 0b0000000000000000 or 0b0000001000000000 indicates that none of
      |  * the setpoint dimensions should be ignored.
      |  *
      |  * If bit 10 is set the floats afx afy afz should be interpreted as force
      |  * instead of acceleration.
      |  *
      |  * Mapping:
      |  * bit 1: x,
      |  * bit 2: y,
      |  * bit 3: z,
      |  * bit 4: vx,
      |  * bit 5: vy,
      |  * bit 6: vz,
      |  * bit 7: ax,
      |  * bit 8: ay,
      |  * bit 9: az,
      |  * bit 10: is force setpoint,
      |  * bit 11: yaw,
      |  * bit 12: yaw rate
      |  * remaining bits unused
      |  *
      |  * Combine bitmasks with bitwise &
      |  *
      |  * Example for position and yaw angle:
      |  * uint16_t type_mask =
      |  *     MAVLINK_MSG_SET_POSITION_TARGET_LOCAL_NED_POSITION &
      |  *     MAVLINK_MSG_SET_POSITION_TARGET_LOCAL_NED_YAW_ANGLE;
      |  */
      |
      |                                                 											// bit number  876543210987654321
      | #define MAVLINK_MSG_SET_POSITION_TARGET_LOCAL_NED_POSITION    			  0b0000 1101 1111 1000
      | #define MAVLINK_MSG_SET_POSITION_TARGET_LOCAL_NED_VELOCITY     	 	  0b0000 1101 1100 0111
      | #define MAVLINK_MSG_SET_POSITION_TARGET_LOCAL_NED_ACCELERATION 	  0b0000 1100 0011 1111
      | #define MAVLINK_MSG_SET_POSITION_TARGET_LOCAL_NED_FORCE        			  0b0000 1110 0011 1111
      | #define MAVLINK_MSG_SET_POSITION_TARGET_LOCAL_NED_YAW_ANGLE   		  0b0000 1001 1111 1111
      | #define MAVLINK_MSG_SET_POSITION_TARGET_LOCAL_NED_YAW_RATE    		  0b0000 0101 1111 1111
  switch_x : Inport
  switch_y : Inport  Port=2
  switch_z : Inport  Port=3
  switch_vx : Inport  Port=4
  switch_vy : Inport  Port=5
  switch_vz : Inport  Port=6
  switch_ax : Inport  Port=7
  switch_ay : Inport  Port=8
  switch_az : Inport  Port=9
  switch_yaw : Inport  Port=10
  switch_yawrate : Inport  Port=11
  (uint16) ALL : Constant  Value=3583  OutDataTypeStr=uint16
  (uint16) DO NOT IGNORE ACEL. X : Constant  Value=3519  OutDataTypeStr=uint16
  (uint16) DO NOT IGNORE ACEL. Y : Constant  Value=3455  OutDataTypeStr=uint16
  (uint16) DO NOT IGNORE ACEL. Z : Constant  Value=3327  OutDataTypeStr=uint16
  (uint16) DO NOT IGNORE VEL. X : Constant  Value=3575  OutDataTypeStr=uint16
  (uint16) DO NOT IGNORE VEL. Y : Constant  Value=3567  OutDataTypeStr=uint16
  (uint16) DO NOT IGNORE VEL. Z : Constant  Value=3551  OutDataTypeStr=uint16
  (uint16) DO NOT IGNORE X1 : Constant  Value=3582  OutDataTypeStr=uint16
  (uint16) DO NOT IGNORE Y1 : Constant  Value=3581  OutDataTypeStr=uint16
  (uint16) DO NOT IGNORE YAW ANGLE : Constant  Value=2559  OutDataTypeStr=uint16
  (uint16) DO NOT IGNORE YAW RATE : Constant  Value=1535  OutDataTypeStr=uint16
  (uint16) DO NOT IGNORE Z3 : Constant  Value=3579  OutDataTypeStr=uint16
  Bitwise AND : simulink/Logic and Bit Operations/Bitwise Operator  logicop=AND  UseBitMask=off  NumInputPorts=11  BitMask=bin2dec('11011001')  BitMaskRealWorld=Stored Integer
  Switch{1..11} (11 alike) : Switch  Criteria=u2 > Threshold
  type_mask : Outport
  wires:
  (uint16) DO NOT IGNORE X1/1 -> Switch1/1
  Switch5/1 -> Bitwise AND/5
  Switch6/1 -> Bitwise AND/6
  Switch1/1 -> Bitwise AND/1
  Switch8/1 -> Bitwise AND/8
  Switch4/1 -> Bitwise AND/4
  Switch7/1 -> Bitwise AND/7
  Switch11/1 -> Bitwise AND/10
  Switch10/1 -> Bitwise AND/11
  Switch9/1 -> Bitwise AND/9
  (uint16) ALL/1 -> Switch8/3, Switch10/3, Switch11/3, Switch9/3, Switch7/3, Switch6/3, Switch5/3, Switch4/3, Switch3/3, Switch2/3, Switch1/3
  Switch2/1 -> Bitwise AND/2
  (uint16) DO NOT IGNORE ACEL. Y/1 -> Switch8/1
  (uint16) DO NOT IGNORE Y1/1 -> Switch2/1
  (uint16) DO NOT IGNORE ACEL. X/1 -> Switch7/1
  (uint16) DO NOT IGNORE VEL. Y/1 -> Switch5/1
  (uint16) DO NOT IGNORE VEL. Z/1 -> Switch6/1
  (uint16) DO NOT IGNORE YAW ANGLE/1 -> Switch11/1
  (uint16) DO NOT IGNORE VEL. X/1 -> Switch4/1
  (uint16) DO NOT IGNORE ACEL. Z/1 -> Switch9/1
  (uint16) DO NOT IGNORE Z3/1 -> Switch3/1
  Switch3/1 -> Bitwise AND/3
  (uint16) DO NOT IGNORE YAW RATE/1 -> Switch10/1
  switch_x/1 -> Switch1/2
  switch_y/1 -> Switch2/2
  switch_z/1 -> Switch3/2
  switch_vx/1 -> Switch4/2
  switch_vy/1 -> Switch5/2
  switch_vz/1 -> Switch6/2
  switch_ax/1 -> Switch7/2
  switch_ay/1 -> Switch8/2
  switch_az/1 -> Switch9/2
  switch_yaw/1 -> Switch11/2
  switch_yawrate/1 -> Switch10/2
  Bitwise AND/1 -> type_mask/1

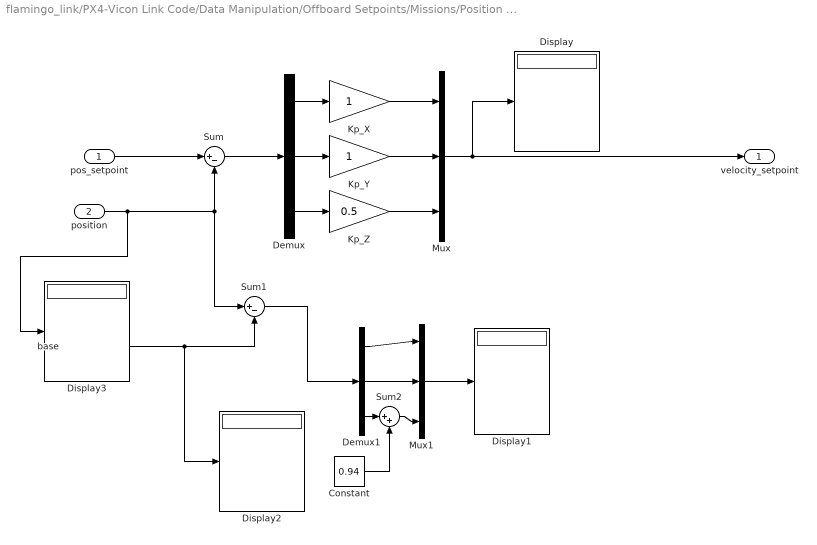
== system flamingo_link/PX4-Vicon Link Code/Data Manipulation/Offboard Setpoints/Missions/Position Controller ==
  pos_setpoint : Inport  PortDimensions=3
  position : Inport  Port=2  PortDimensions=3
  "base " : Inport  Port=3  PortDimensions=3
  Constant : Constant  Value=0.94
  Demux : Demux  Outputs=3
  Demux1 : Demux  Outputs=3
  Display{,1..3} (4 alike) : Display
  Kp_X : Gain
  Kp_Y : Gain
  Kp_Z : Gain  Gain=0.5
  Mux : Mux  Inputs=3
  Mux1 : Mux  Inputs=3
  Sum : Sum  Inputs=|+-
  Sum1 : Sum  Inputs=|+-
  Sum2 : Sum  Inputs=|++
  velocity_setpoint : Outport  PortDimensions=3
  wires:
  Sum/1 -> Demux/1
  pos_setpoint/1 -> Sum/1
  Mux/1 -> Display/1, velocity_setpoint/1
  Demux/1 -> Kp_X/1
  Demux/2 -> Kp_Y/1
  Demux/3 -> Kp_Z/1
  Kp_X/1 -> Mux/1
  Kp_Y/1 -> Mux/2
  Kp_Z/1 -> Mux/3
  position/1 -> Display3/1, Sum/2, Sum1/1
  "base "/1 -> Display2/1, Sum1/2
  Sum1/1 -> Demux1/1
  Demux1/1 -> Mux1/1
  Demux1/2 -> Mux1/2
  Demux1/3 -> Sum2/1
  Sum2/1 -> Mux1/3
  Constant/1 -> Sum2/2
  Mux1/1 -> Display1/1

== system flamingo_link/PX4-Vicon Link Code/Data Manipulation/Offboard Setpoints/Missions/Switch Case Action Subsystem ==
  In1 : Inport
  Action Port : ActionPort  ActionPortLabel=case [ 0 ]:
  Out1 : Outport
  wires:
  In1/1 -> Out1/1

== system flamingo_link/PX4-Vicon Link Code/Data Manipulation/Offboard Setpoints/Missions/Switch Case Action Subsystem1 ==
  In1 : Inport
  Action Port : ActionPort  ActionPortLabel=case [ 1 ]:
  Out1 : Outport
  wires:
  In1/1 -> Out1/1

== system flamingo_link/PX4-Vicon Link Code/Data Manipulation/Offboard Setpoints/Missions/Switch Case Action Subsystem2 ==
  In1 : Inport
  Action Port : ActionPort  ActionPortLabel=case [ 2 ]:
  Out1 : Outport
  wires:
  In1/1 -> Out1/1

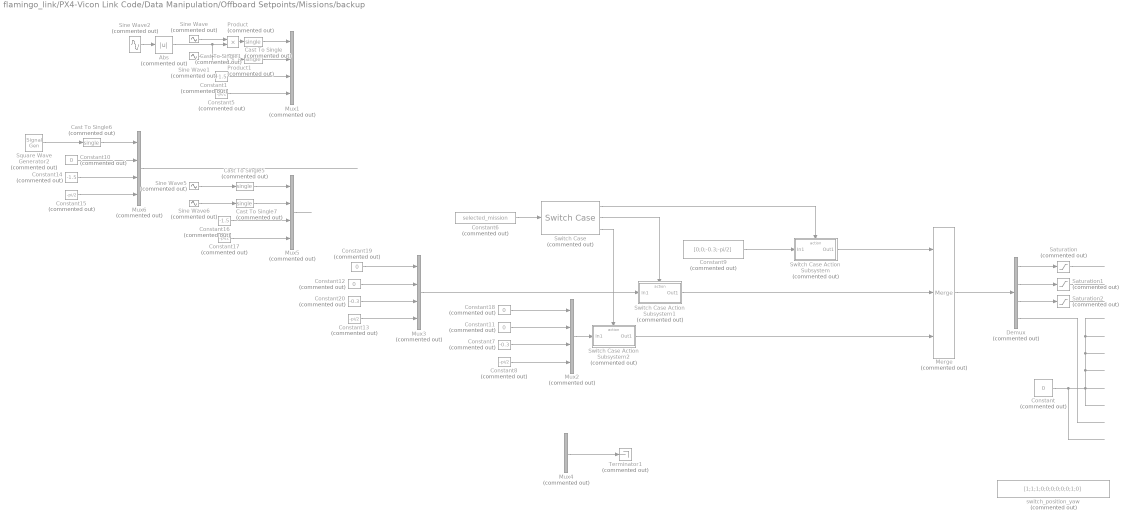
== system flamingo_link/PX4-Vicon Link Code/Data Manipulation/Offboard Setpoints/Missions/backup ==
  Abs : Abs  Commented=on
  Cast To Single{,1,5..7} (5 alike) : DataTypeConversion  Commented=on  OutDataTypeStr=single
  Constant{,10..12,18..19} (6 alike) : Constant  Commented=on  Value=0  OutDataTypeStr=single
  Constant1 : Constant  Commented=on  Value=-1.5  OutDataTypeStr=single
  Constant{5,8,13,15,17} (5 alike) : Constant  Commented=on  Value=-pi/2  OutDataTypeStr=single
  Constant14 : Constant  Commented=on  Value=-1.5  OutDataTypeStr=single
  Constant16 : Constant  Commented=on  Value=-1.5  OutDataTypeStr=single
  Constant20 : Constant  Commented=on  Value=-0.3  OutDataTypeStr=single
  Constant6 : Constant  Commented=on  Value=selected_mission
  Constant7 : Constant  Commented=on  Value=-0.3  OutDataTypeStr=single
  Constant9 : Constant  Commented=on  Value=[0;0;-0.3;-pi/2]  OutDataTypeStr=single
  Demux : Demux  Commented=on
  Merge : Merge  Commented=on  Inputs=3
  Mux{1..3,5..6} (5 alike) : Mux  Commented=on
  Mux4 : Mux  Commented=on  Inputs=2
  Product : Product  Commented=on
  Product1 : Product  Commented=on
  Saturation : Saturate  Commented=on  UpperLimit=2.5  LowerLimit=-2.5
  Saturation1 : Saturate  Commented=on  UpperLimit=2.5  LowerLimit=-2.5
  Saturation2 : Saturate  Commented=on  UpperLimit=0  LowerLimit=-2.5
  Sine Wave : Sin  Commented=on  Frequency=0.5  SampleTime=0
  Sine Wave1 : Sin  Commented=on  Frequency=0.5  Phase=pi/2  SampleTime=0
  Sine Wave2 : Sin  Commented=on  Amplitude=2.5  SampleTime=0
  Sine Wave5 : Sin  Commented=on  Amplitude=1.5  Frequency=0.3  SampleTime=0
  Sine Wave6 : Sin  Commented=on  Amplitude=1.5  Frequency=0.3  Phase=pi/2  SampleTime=0
  Square Wave Generator2 : SignalGenerator  Commented=on  WaveForm=square  Amplitude=1.5  Frequency=0.35  Units=rad/sec
  Switch Case : SwitchCase  Commented=on  CaseConditions={0,1,2}  ShowDefaultCase=off
  Switch Case Action Subsystem : Subsystem  Commented=on  TreatAsAtomicUnit=on
  Switch Case Action Subsystem1 : Subsystem  Commented=on  TreatAsAtomicUnit=on
  Switch Case Action Subsystem2 : Subsystem  Commented=on  TreatAsAtomicUnit=on
  Terminator1 : Terminator  Commented=on
  switch_position_yaw : Constant  Commented=on  Value=[1;1;1;0;0;0;0;0;0;1;0]  OutDataTypeStr=single
  wires:
  Saturation/1 -> ?
  Cast To Single/1 -> Mux1/1
  Cast To Single1/1 -> Mux1/2
  Constant5/1 -> Mux1/4
  Switch Case Action Subsystem1/1(Out1) -> Merge/2
  Sine Wave1/1 -> Product1/1
  Demux/1 -> Saturation/1
  Constant1/1 -> Mux1/3
  Constant/1 -> ?
  Sine Wave/1 -> Product/1
  Demux/4 -> ?
  Switch Case/1 -> Switch Case Action Subsystem/Action
  Abs/1 -> Product1/2, Product/2
  Product1/1 -> Cast To Single1/1
  Saturation2/1 -> ?
  Constant6/1 -> Switch Case/1
  Sine Wave2/1 -> Abs/1
  Mux4/1 -> Terminator1/1
  Demux/3 -> Saturation2/1
  Constant16/1 -> Mux5/3
  Constant12/1 -> Mux3/2
  Constant11/1 -> Mux2/2
  Constant20/1 -> Mux3/3
  Mux5/1 -> ?
  Constant14/1 -> Mux6/3
  Constant19/1 -> Mux3/1
  Cast To Single6/1 -> Mux6/1
  Sine Wave5/1 -> Cast To Single5/1
  Constant18/1 -> Mux2/1
  Sine Wave6/1 -> Cast To Single7/1
  Constant15/1 -> Mux6/4
  Demux/2 -> Saturation1/1
  Constant9/1 -> Switch Case Action Subsystem/1(In1)
  Switch Case Action Subsystem2/1(Out1) -> Merge/3
  Switch Case Action Subsystem/1(Out1) -> Merge/1
  Cast To Single7/1 -> Mux5/2
  Mux6/1 -> ?
  Constant7/1 -> Mux2/3
  Mux2/1 -> Switch Case Action Subsystem2/1(In1)
  Constant10/1 -> Mux6/2
  Switch Case/2 -> Switch Case Action Subsystem1/Action
  Square Wave Generator2/1 -> Cast To Single6/1
  Merge/1 -> Demux/1
  Mux3/1 -> Switch Case Action Subsystem1/1(In1)
  Cast To Single5/1 -> Mux5/1
  Constant13/1 -> Mux3/4
  Switch Case/3 -> Switch Case Action Subsystem2/Action
  Saturation1/1 -> ?
  Constant17/1 -> Mux5/4
  Product/1 -> Cast To Single/1
  Constant8/1 -> Mux2/4

== system flamingo_link/PX4-Vicon Link Code/Data Manipulation/Offboard Setpoints/Missions/backup/Switch Case Action Subsystem ==
  In1 : Inport
  Action Port : ActionPort  ActionPortLabel=case [ 0 ]:
  Out1 : Outport
  wires:
  In1/1 -> Out1/1

== system flamingo_link/PX4-Vicon Link Code/Data Manipulation/Offboard Setpoints/Missions/backup/Switch Case Action Subsystem1 ==
  In1 : Inport
  Action Port : ActionPort  ActionPortLabel=case [ 1 ]:
  Out1 : Outport
  wires:
  In1/1 -> Out1/1

== system flamingo_link/PX4-Vicon Link Code/Data Manipulation/Offboard Setpoints/Missions/backup/Switch Case Action Subsystem2 ==
  In1 : Inport
  Action Port : ActionPort  ActionPortLabel=case [ 2 ]:
  Out1 : Outport
  wires:
  In1/1 -> Out1/1

== stateflow chart flamingo_link/PX4-Vicon Link Code/Data Manipulation/Offboard Setpoints/Mode Logic ==
  state ModesLogic [parallel]
    settings: executionOrder=1
    (history)
    state Land
      set_switch_out = [1;1;1;0;0;0;0;0;0;1;0];
      en: p = position;
      y = yaw;
      takeoff_detected = 0;
      du: setpoints_out = [p(1);p(2);0;0;0;0;0;0;0;y;0];
      status = 1;
    state Takeoff
      set_switch_out = [1;1;1;0;0;0;0;0;0;1;0];
      en: p = position;
      y = yaw;
      du: setpoints_out = [p(1);p(2);-1.5;0;0;0;0;0;0;y;0];
      status = 2;
      if(duration(abs(-1.5-position(3)) <= 0.1) > 3)
      takeoff_detected = 1;
      end
    state Hold
      set_switch_out = [1;1;1;0;0;0;0;0;0;1;0];
      en: p = position;
      y = yaw;
      takeoff_detected = 0;
      du: status = 3;
      setpoints_out = [p(1);p(2);p(3);0;0;0;0;0;0;y;0]
    state Return
      set_switch_out = [1;1;1;0;0;0;0;0;0;1;0];
      setpoints_out = single([0;0;-1.5;0;0;0;0;0;0;-pi/2;0]);
      du: status = 4;
      if((abs(position(1)) < 2.6) && (abs(position(2)) < 2.6) && (abs(position(3)) < 2.6))
      fence_detected = 0;
      end
    state Mission
      set_switch_out = mission_switch_in;
      setpoints_out = mission_setpoints_in;
      en: takeoff_detected = 0;
      du: status = 5;
      if((abs(position(1)) >= 2.6) || (abs(position(2)) >= 2.6) || (abs(position(3)) >= 2.6))
      fence_detected = 1;
      end
    state Direct
      set_switch_out = set_switch_in;
      setpoints_out = setpoints_in;
      en: takeoff_detected = 0;
      du: status = 6;
      if((abs(position(1)) >= 2.6) || (abs(position(2)) >= 2.6) || (abs(position(3)) >= 2.6))
      fence_detected = 1;
      end
    Return -> Land [order 2] : [land_com == 1]
    Hold -> Land [order 1] : [land_com == 1]
    (default) -> Land : {fence_detected = 0;}
    Takeoff -> Hold [order 3] : [((hold_com == 1) ||  (takeoff_detected == 1))]
    Land -> Takeoff [order 1] : [takeoff_com == 1]
    Return -> Hold [order 3] : [hold_com == 1]
    Takeoff -> Land [order 2] : [land_com == 1]
    Hold -> Return [order 2] : [return_com == 1]
    Direct -> Land [order 3] : [land_com == 1]
    Land -> Direct [order 3] : [direct_com == 1]
    Takeoff -> Direct [order 4] : [direct_com == 1]
    Takeoff -> Mission [order 1] : [mission_com == 1]
    Hold -> Mission [order 3] : [mission_com == 1]
    Hold -> Direct [order 4] : [direct_com == 1]
    Direct -> Hold [order 4] : [((hold_com == 1) || (fence_detected == 1))]
    Mission -> Hold [order 3] : [((hold_com == 1) || (fence_detected == 1))]
    Return -> Direct [order 4] : [direct_com == 1]
    Mission -> Return [order 2] : [return_com == 1]
    Direct -> Return [order 1] : [return_com == 1]
    Return -> Mission [order 1] : [mission_com == 1]
    Mission -> Land [order 1] : [land_com == 1]
    Land -> Mission [order 2] : [mission_com == 1]
    Mission -> Direct [order 4] : [direct_com == 1]
    Direct -> Mission [order 2] : [mission_com == 1]
  data: setpoints_in input single size=11; set_switch_in input single size=11; return_com input; takeoff_com input; mission_com input; hold_com input; land_com input; direct_com input; setpoints_out output single size=11; set_switch_out output single size=11; position input size=3; p local size=3; y local size=1; yaw input size=1; takeoff_detected local size=1; fence_detected local; mission_switch_in input; mission_setpoints_in input; status output
